simulink model "simu2"  (R2019b)
settings: Solver=VariableStepAuto  StartTime=0.0  StopTime=10.0  RelTol=1e-3
settings Model: Creator=Admin  LastModifiedBy=Admin

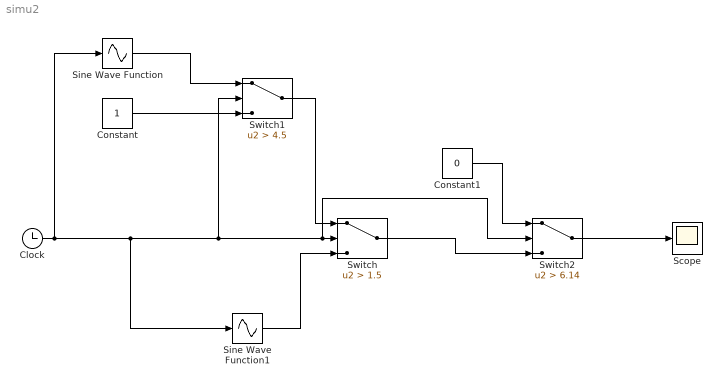
== system simu2 ==
  Clock : Clock
  Constant : Constant
  Constant1 : Constant  Value=0
  Scope : Scope
  Sine Wave Function : Sin  TimeSource=Use external signal  Phase=-3  SampleTime=0
  Sine Wave Function1 : Sin  TimeSource=Use external signal  SampleTime=0
  Switch : Switch  Criteria=u2 > Threshold  Threshold=1.5
  Switch1 : Switch  Criteria=u2 > Threshold  Threshold=4.5
  Switch2 : Switch  Criteria=u2 > Threshold  Threshold=6.14
  wires:
  Clock/1 -> Switch1/2, Switch2/2, Switch/2, Sine Wave Function1/1, Sine Wave Function/1
  Sine Wave Function1/1 -> Switch/3
  Switch1/1 -> Switch/1
  Sine Wave Function/1 -> Switch1/1
  Constant/1 -> Switch1/3
  Switch/1 -> Switch2/3
  Constant1/1 -> Switch2/1
  Switch2/1 -> Scope/1
